simulink model "TwinCAT_modules"  (R2017b)
settings: Solver=FixedStepAuto  StartTime=0.0  StopTime=240  FixedStep=0.005  RelTol=1e-3
undefined symbols (not defined in the file or in its folder): PolePlacer
libraries: aerolibconvert2 x1, simulink x1, cstblocks x1
settings Model: Creator=motionlab  LastModifiedBy=motionlab
settings OptimizationCC: LocalBlockOutputs=off
settings RTWCC: SystemTargetFile=TwinCAT.tlc  GenCodeOnly=on  MakeCommand=make_tct  TemplateMakefile=tct_msbuild.tmf  Description=TwinCAT Target  GenerateReport=on  TargetLang=C++  CheckMdlBeforeBuild=Warning
settings STFCustomTargetCC: TargetLangStandard=C++03 (ISO)  CompOptLevelCompliant=on  MATLABClassNameForMDSCustomization=Simulink.SoftwareTarget.TargetSpecificTriggerConfigurationBase  SystemTargetFile=TwinCAT.tlc

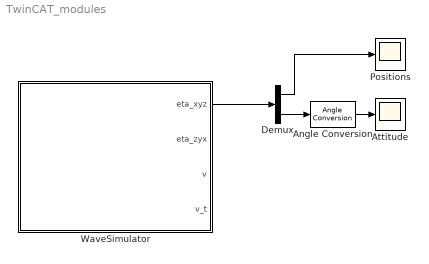
== system TwinCAT_modules ==
  Angle Conversion : aerolibconvert2/Angle Conversion  IU=rad  OU=deg
  Attitude : Scope
  Demux : Demux  Outputs=2
  Positions : Scope
  WaveSimulator : Subsystem
  wires:
  Angle Conversion/1 -> Attitude/1
  Demux/1 -> Positions/1
  Demux/2 -> Angle Conversion/1
  WaveSimulator/1(eta_xyz) -> Demux/1

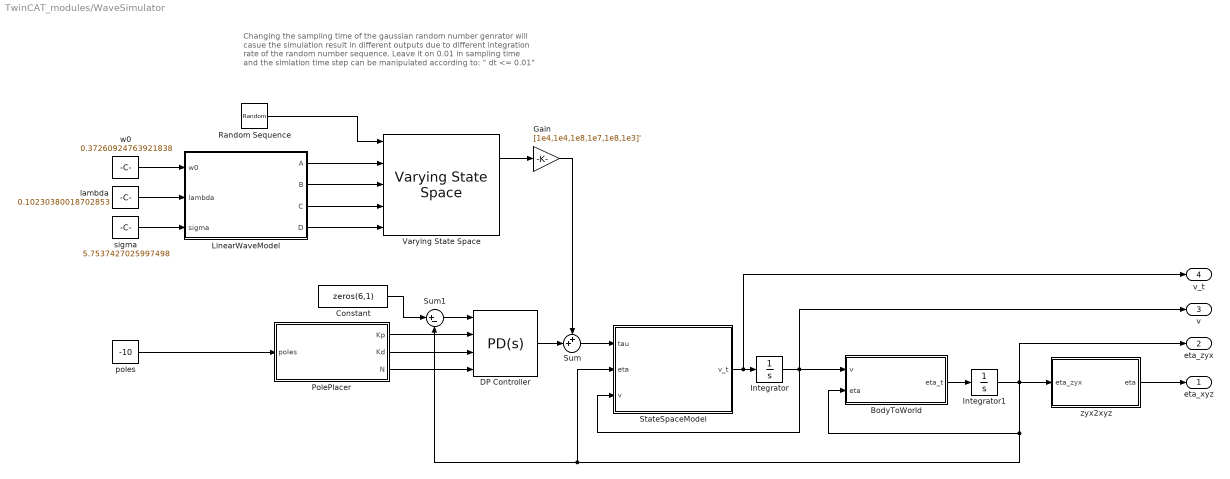
== system TwinCAT_modules/WaveSimulator ==
  note: Changing the sampling time of the gaussian random number genrator will casue the simulation result in different outputs due to different integration rate of the random number sequence. Leave it on 0.01 in sampling time and the simlation time step can be manipulated according to: " dt <= 0.01"
  BodyToWorld : MATLAB Function  TreatAsAtomicUnit=on
  Constant : Constant  Value=zeros(6,1)
  DP Controller : simulink/Continuous/PID Controller  Controller=PD  TimeDomain=Continuous-time  SampleTime=-1  IntegratorMethod=Forward Euler  FilterMethod=Forward Euler  Form=Parallel  UseFilter=on  ControllerParametersSource=external  P=PolePlacer(3, 100, 'P')  I=1  D=PolePlacer(3, 100, 'D')  N=100  InitialConditionSource=internal  InitialConditionForIntegrator=0  InitialConditionForFilter=0  ExternalReset=none  LimitOutput=off  UpperSaturationLimit=inf  LowerSaturationLimit=-inf  LinearizeAsGain=on  AntiWindupMode=none  Kb=1  TrackingMode=off  Kt=1  PParamMin=[]  PParamMax=[]  IParamMin=[]  IParamMax=[]  DParamMin=[]  DParamMax=[]  NParamMin=[]  NParamMax=[]  KbParamMin=[]  KbParamMax=[]  KtParamMin=[]  KtParamMax=[]  POutMin=[]  POutMax=[]  IOutMin=[]  IOutMax=[]  DOutMin=[]  DOutMax=[]  NOutMin=[]  NOutMax=[]  KbOutMin=[]  KbOutMax=[]  KtOutMin=[]  KtOutMax=[]  IntegratorOutMin=[]  IntegratorOutMax=[]  FilterOutMin=[]  FilterOutMax=[]  SumOutMin=[]  SumOutMax=[]  SumI1OutMin=[]  SumI1OutMax=[]  SumI2OutMin=[]  SumI2OutMax=[]  SumI3OutMin=[]  SumI3OutMax=[]  SumDOutMin=[]  SumDOutMax=[]  SaturationOutMin=[]  SaturationOutMax=[]  IntegratorContinuousStateAttributes=''  IntegratorStateMustResolveToSignalObject=off  IntegratorRTWStateStorageClass=Auto  FilterContinuousStateAttributes=''  FilterStateMustResolveToSignalObject=off  FilterRTWStateStorageClass=Auto  DifferentiatorICPrevScaledInput=0  DifferentiatorOutMin=[]  DifferentiatorOutMax=[]  InitialConditionSetting=State (most efficient)  FilterDiffOutCoefMin=[]  FilterDiffOutCoefMax=[]  SumDenOutMin=[]  SumDenOutMax=[]  SumNumOutMin=[]  SumNumOutMax=[]  ReciprocalOutMin=[]  ReciprocalOutMax=[]  DivideOutMin=[]  DivideOutMax=[]  TunerSelectOption=Transfer Function Based (PID Tuner App)
  Gain : Gain  Gain=[1e4,1e4,1e8,1e7,1e8,1e3]'
  Integrator : Integrator  InitialCondition=zeros(6,1)
  Integrator1 : Integrator  InitialCondition=zeros(6,1)
  LinearWaveModel : MATLAB Function  TreatAsAtomicUnit=on  SystemSampleTime=1
  PolePlacer : MATLAB Function  TreatAsAtomicUnit=on  SystemSampleTime=1
  Random Sequence : RandomNumber  Mean=zeros(6,1)  Variance=ones(6,1)  Seed=[0,20,500,9000,400,200]  SampleTime=0.01
  StateSpaceModel : MATLAB Function  TreatAsAtomicUnit=on
  Sum : Sum  Inputs=++|
  Sum1 : Sum  Inputs=|+-
  Varying State Space : cstblocks/Linear Parameter Varying/Varying State Space  x0=zeros(12,1)'  xNames=''  OutputX=on  OutputDX=off
      settings: SourceProductName=Control System Toolbox
  lambda : Constant  Value=0.10230380018702853
  poles : Constant  Value=-10
  sigma : Constant  Value=5.7537427025997498
  w0 : Constant  Value=0.37260924763921838
  zyx2xyz : MATLAB Function  TreatAsAtomicUnit=on
  eta_xyz : Outport
  eta_zyx : Outport  Port=2
  v : Outport  Port=3
  v_t : Outport  Port=4
  wires:
  Random Sequence/1 -> Varying State Space/1
  DP Controller/1 -> Sum/2
  StateSpaceModel/1(v_t) -> v_t/1, Integrator/1
  BodyToWorld/1(eta_t) -> Integrator1/1
  Sum1/1 -> DP Controller/1
  Sum/1 -> StateSpaceModel/1(tau)
  Integrator/1 -> v/1, BodyToWorld/1(v), StateSpaceModel/3(v)
  PolePlacer/2(Kd) -> DP Controller/3
  PolePlacer/3(N) -> DP Controller/4
  PolePlacer/1(Kp) -> DP Controller/2
  LinearWaveModel/1(A) -> Varying State Space/2
  LinearWaveModel/3(C) -> Varying State Space/4
  LinearWaveModel/2(B) -> Varying State Space/3
  LinearWaveModel/4(D) -> Varying State Space/5
  Varying State Space/1 -> Gain/1
  Integrator1/1 -> eta_zyx/1, BodyToWorld/2(eta), Sum1/2, StateSpaceModel/2(eta), zyx2xyz/1(eta_zyx)
  Gain/1 -> Sum/1
  Constant/1 -> Sum1/1
  w0/1 -> LinearWaveModel/1(w0)
  lambda/1 -> LinearWaveModel/2(lambda)
  sigma/1 -> LinearWaveModel/3(sigma)
  poles/1 -> PolePlacer/1(poles)
  zyx2xyz/1(eta) -> eta_xyz/1

== matlab function TwinCAT_modules/WaveSimulator/BodyToWorld ==
  data: v input; eta_t output; eta input
function eta_t  = BodyToWorld(v, eta)

% Vessel kinemamtics
phi = eta(4:6);

J = eye(6);

% Fossen's hydrodynamics jacobian version
J(1:3,1:3) = Rz(phi(3))*Ry(phi(2))*Rx(phi(1));
J(4:6,4:6) = Tphi(phi, 'zyx');

% {b} -> {n}
eta_t = J*v;
    
end

== matlab function TwinCAT_modules/WaveSimulator/StateSpaceModel ==
  data: tau input; eta input; v_t output; v input
function v_t = StateSpaceModel(tau, eta, v)

    % Load data from mss file
    data = coder.load('supply.mat');

    v_t = zeros(6,1);
    
    v_t = data.supply.Minv*(tau - data.supply.D*v - data.supply.G*eta);

end

== matlab function TwinCAT_modules/WaveSimulator/PolePlacer ==
  data: poles input; Kp output; Kd output; N output
function [Kp, Kd, N] = PolePlacer(poles)
    
    % Load estimated 1st order model data for surge, sway and yaw motion
    data = coder.load('step.mat');
    
    % 1st order plant paramaters
    Kss = [
            data.step.surge.Kss,
            data.step.sway.Kss,
            data.step.yaw.Kss
        ];
    
    tau = [
            data.step.surge.tau,
            data.step.sway.tau,
            data.step.yaw.tau
        ];
    
    Kp = zeros(6,1);
    Kd = zeros(6,1);
    
    % Calculate gains analytically 
    N = 100;
    
    poles = abs(poles);
    
    max_placement = 30.0;
    if poles >= max_placement
        poles = max_placement;
    end
    
    Kp(1) = (tau(1)*poles^2 - N)/(Kss(1)*N);
    Kp(2) = (tau(2)*poles^2 - N)/(Kss(2)*N);
    Kp(6) = (tau(3)*poles^2 - N)/(Kss(3)*N);
    
    Kd(1) = (2*tau(1)*poles - 1 - Kp(1)*Kss(1) - tau(1)*N)/(Kss(1)*N);
    Kd(2) = (2*tau(2)*poles - 1 - Kp(2)*Kss(2) - tau(2)*N)/(Kss(2)*N);
    Kd(6) = (2*tau(3)*poles - 1 - Kp(6)*Kss(3) - tau(3)*N)/(Kss(3)*N);
    
    Kp = abs(Kp);
    Kd = abs(Kd);
end

== matlab function TwinCAT_modules/WaveSimulator/LinearWaveModel ==
  data: w0 input; A output; B output; C output; lambda input; sigma input; D output
function [A, B, C, D] = LinearWaveModel(w0, lambda, sigma)
    
    % p. 216-220 in "Fossen, T. I. (2011). Handbook of Marine Craft
    % Hydrodynamics and Motion Control"
    
    
    % Linearized wave spectrum model matrices
    
    Kw = abs(2*lambda*w0*sigma);
    
    % A
    a = [    0,                 1;
         -w0^2, -2*abs(lambda*w0)];
    
    A = blkdiag(a,a,a,a,a,a);
    
    % B
    b = [0; Kw];
    
    B = blkdiag(b,b,b,b,b,b);
    
    % C
    c = [0, 1];
    
    C = blkdiag(c,c,c,c,c,c);
    
    % D
    D = zeros(6,6);
    
end

== matlab function TwinCAT_modules/WaveSimulator/zyx2xyz ==
  data: eta output; eta_zyx input
function eta  = zyx2xyz(eta_zyx)

phi = eta_zyx(4:6);

eta = zeros(6,1);
eta(1:3) = eta_zyx(1:3);

% Maple code
t1 = sin(phi(1));
t2 = cos(phi(3));
t3 = cos(phi(1));
t4 = sin(phi(2));
t5 = sin(phi(3));
t6 = t3 * t5;
t7 = t1 * t2;
t8 = cos(phi(2));

eta(4) = atan2((-t6 * t4 + t7),(t3 * t8));
eta(5) = asin(t3 * t4 * t2 + t1 * t5);
eta(6) = atan2((-t7 * t4 + t6),( t2 * t8));

end
